simulink model "simulink_implementation_usingbuffer"  (R2019b)
settings: Solver=FixedStepDiscrete  StartTime=0.0  StopTime=timetorun  RelTol=1e-3
undefined symbols (not defined in the file): buffer_ratio, dsp_slices, sample_rate, v_in
libraries: hdlsllib x2, dspsrcs4 x2
settings Model: DataTypeOverride=Off  Creator=ian  LastModifiedBy=ian
settings DataIOCC: LimitDataPoints=on  SaveOutput=off  SaveTime=off
settings OptimizationCC: BlockReduction=off  ConditionallyExecuteInputs=off  DefaultParameterBehavior=Inlined  LifeSpan=inf
settings DebuggingCC: AlgebraicLoopMsg=error  SingleTaskRateTransMsg=error  AllowSymbolicDim=off  StrictBusMsg=ErrorOnBusTreatedAsVector  SFUnexpectedBacktrackingDiag=warning  SFNoUnconditionalDefaultTransitionDiag=warning  SFExecutionAtInitializationDiag=none  ArithmeticOperatorsInVariantConditions=warning
settings HardwareCC: ProdBitPerPointer=32  ProdBitPerSizeT=32  ProdBitPerPtrDiffT=32  ProdLargestAtomicFloat=None  ProdIntDivRoundTo=Undefined  ProdEndianess=Unspecified  ProdWordSize=32  ProdHWDeviceType=ASIC/FPGA->ASIC/FPGA  TargetBitPerPointer=64  TargetBitPerSizeT=64  TargetBitPerPtrDiffT=64  TargetLongLongMode=on  TargetIntDivRoundTo=Zero  TargetEndianess=LittleEndian  TargetWordSize=64  TargetHWDeviceType=Custom Processor->MATLAB Host Computer  ProdEqTarget=off
settings SFSimCC: SimUseLocalCustomCode=off  CustomCodeUndefinedFunction=UseInterfaceOnly
settings RTWCC: RTWUseLocalCustomCode=off
settings CodeAppCC: StateflowObjectComments=on
settings GRTTargetCC: TargetLangStandard=C89/C90 (ANSI)  GeneratePreprocessorConditionals=Disable all
settings ConfigComp: CovScope=ReferencedModels  CovMetricSettings=dw  CovHtmlReporting=on  CovSaveCumulativeToWorkspaceVar=on  CovSaveSingleToWorkspaceVar=on  CovExternalEMLEnable=off  CovSFcnEnable=off

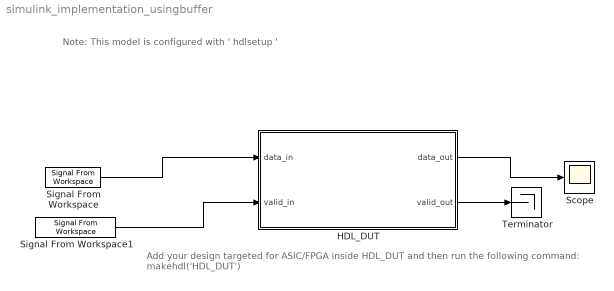
== system simulink_implementation_usingbuffer ==
  note: Note: This model is configured with ' hdlsetup '
  note: Add your design targeted for ASIC/FPGA inside HDL_DUT and then run the following command:
      | makehdl('HDL_DUT')
  HDL_DUT : Subsystem
  Scope : Scope
  Signal From Workspace : dspsrcs4/Signal From Workspace  X=v_in  Ts=sample_rate  nsamps=dsp_slices  OutputAfterFinalValue=Setting to zero  ignoreOrWarnInputAndFrameLengths=off  OutputFrames=off
  Signal From Workspace1 : dspsrcs4/Signal From Workspace  X=true(size(v_in))  Ts=sample_rate  nsamps=1  OutputAfterFinalValue=Setting to zero  ignoreOrWarnInputAndFrameLengths=off  OutputFrames=off
  Terminator : Terminator
  wires:
  HDL_DUT/1(data_out) -> Scope/1
  Signal From Workspace/1 -> HDL_DUT/1(data_in)
  Signal From Workspace1/1 -> HDL_DUT/2(valid_in)
  HDL_DUT/2(valid_out) -> Terminator/1

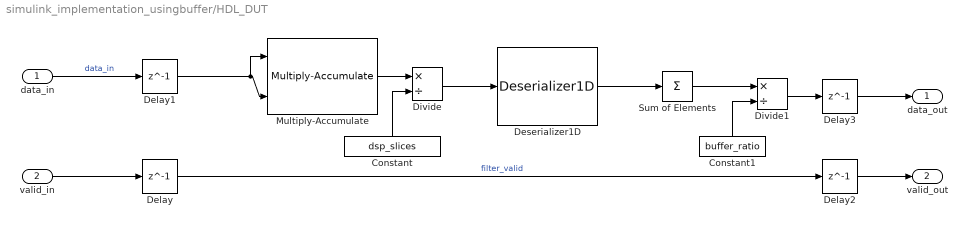
== system simulink_implementation_usingbuffer/HDL_DUT ==
  data_in : Inport
  valid_in : Inport  Port=2
  Constant : Constant  Value=dsp_slices  SampleTime=-1
  Constant1 : Constant  Value=buffer_ratio  SampleTime=-1
  Delay{,1..3} (4 alike) : Delay  DelayLength=1
  Deserializer1D : hdlsllib/HDL Operations/Deserializer1D  Ratio=buffer_ratio  IdleCycles=0  InitialCondition=0  startIn=off  validIn=off  validOut=off  inputDataDimensions=-1  inputSampleTime=-1  inputSignalType=auto
      settings: SourceProductName=Simulink  SourceProductBaseCode=SL
  Divide : Product  Inputs=*/  SaturateOnIntegerOverflow=on  RndMeth=Zero
  Divide1 : Product  Inputs=*/
  Multiply-Accumulate : hdlsllib/HDL Operations/Multiply-Accumulate  opMode=Vector  initValueSetting=Dialog  initValue=0  initValueSetting2=Dialog  initValue2=0  initValueSetting3=Dialog  initValue3=0  num_samples=5  RndMeth=Nearest  RndMeth2=Floor  RndMeth3=Floor  datatype2=Inherit: Inherit via back propagation  datatype3=fixdt(1,16,0)  validOut=on  endInandOut=on  startOut=on  countOut=on  dim=-1  DoSatur=off  parallel=off
      settings: SourceProductName=Simulink  SourceProductBaseCode=SL
  Sum of Elements : Sum  Inputs=+
  data_out : Outport  VectorParamsAs1DForOutWhenUnconnected=off
  valid_out : Outport  Port=2  VectorParamsAs1DForOutWhenUnconnected=off
  wires:
  data_in/1 -> Delay1/1  "data_in"
  Multiply-Accumulate/1 -> Divide/1
  Constant/1 -> Divide/2
  Divide/1 -> Deserializer1D/1
  Deserializer1D/1 -> Sum of Elements/1
  Divide1/1 -> Delay3/1
  Sum of Elements/1 -> Divide1/1
  Constant1/1 -> Divide1/2
  valid_in/1 -> Delay/1
  Delay1/1 -> Multiply-Accumulate/1, Multiply-Accumulate/2
  Delay/1 -> Delay2/1  "filter_valid"
  Delay3/1 -> data_out/1
  Delay2/1 -> valid_out/1
